simulink model "Simulink_Assignment2"  (R2020a)
settings: Solver=FixedStepAuto  StartTime=0.0  StopTime=10  FixedStep=1e-3  RelTol=1e-3  EnableMultiTasking=on
undefined symbols (not defined in the file): A0, A1, D0, D1, D10, D11, D12, D13, D2, D3, D4, D5, D6, D7, D8, D9, magnitude, PTA0, PTA1, PTA2, PTB2, PTB23, PTB3, PTB9, PTC16, PTC17, PTC2, PTC3, PTC4, PTD0, PTD1, PTD2, PTD3
libraries: frdmk64flib x19, etargetslib x8
settings Model: ExtModeTrigDuration=5  Creator=ryanb  LastModifiedBy=hunte
settings OptimizationCC: EnhancedBackFolding=on  PassReuseOutputArgsAs=Individual arguments  ZeroExternalMemoryAtStartup=off  ZeroInternalMemoryAtStartup=off  MaxStackSize=64  OptimizeBlockOrder=speed  DifferentSizesBufferReuse=on  OptimizationCustomize=off  EfficientTunableParamExpr=on
settings DebuggingCC: ParameterTunabilityLossMsg=error  UnconnectedInputMsg=none  UnconnectedOutputMsg=none  UnconnectedLineMsg=none
settings HardwareCC: ProdBitPerPointer=32  ProdBitPerSizeT=32  ProdBitPerPtrDiffT=32  ProdLargestAtomicInteger=Long  ProdLargestAtomicFloat=Double  ProdWordSize=32  ProdHWDeviceType=ARM Compatible->ARM Cortex
settings ModelReferenceCC: EnableRefExpFcnMdlSchedulingChecks=off
settings SFSimCC: MATLABDynamicMemAlloc=off
settings RTWCC: SystemTargetFile=ert.tlc  HardwareBoard=NXP FRDM-K64F  TemplateMakefile=ert_default_tmf  Toolchain=GNU Tools for ARM Embedded Processors
settings CodeAppCC: ForceParamTrailComments=on  IgnoreCustomStorageClasses=off  OperatorAnnotations=on  SimulinkDataObjDesc=on  SFDataObjDesc=on  InsertBlockDesc=on
settings ERTTargetCC: ExtModeTransport=4  ExtModeMexFile=sendToCommService

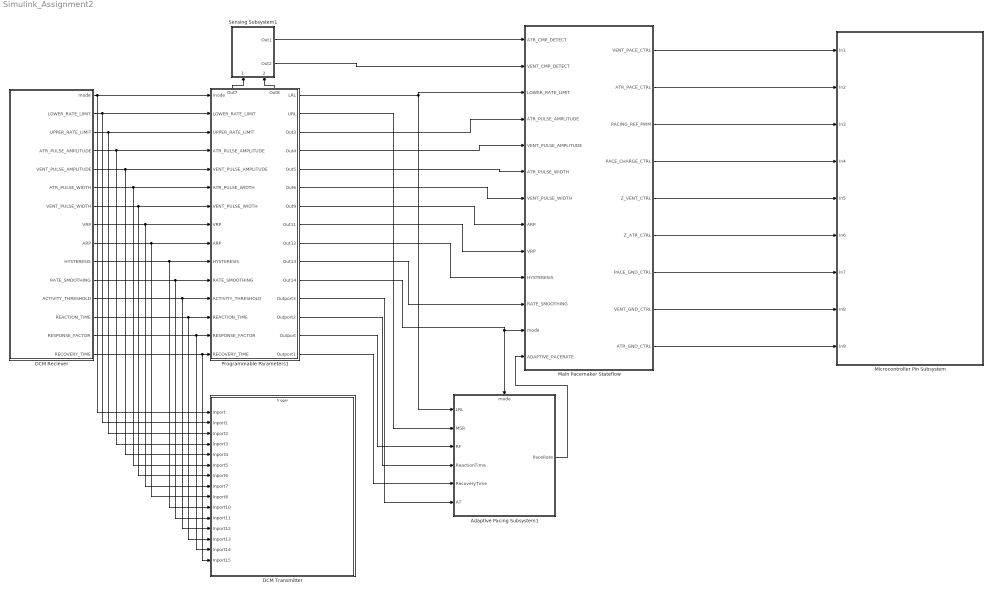
== system Simulink_Assignment2 ==
  Adaptive Pacing Subsystem1 : Subsystem
      settings: PortSchema="{\"entries\":[{\"content\":{\"sides\":[{\"content\":{\"connectorIds\":[\"In1\",\"In2\",\"In3\",\"In4\",\"In5\",\"In6\"]},\"type\":\"ConnectorPlacement.EquallySpacedRectSide\",\"uuid\":\"61dbb7e9-2003-4a43-93b8-10f5910df485\"},{\"content\":{\"connectorIds\":[\"Out1\"],\"side\":\"RIGHT\"},\"type\":\"ConnectorPlacement.EquallySpacedRectSide\",\"uuid\":\"cbb870a5-2f34-4900-b14d-ede4f510cea2\"},{\"content\":{\"connectorIds\":[\"In7\"],\"side\":\"TOP\"},\"type\":\"ConnectorPlacement.EquallySpacedRectSide\",\"uuid\":\"f277726d-3108-4a56-8fdd-1a2c1e5413e5\"}]},\"type\":\"ConnectorPlacement.EquallySpacedConnector\",\"uuid\":\"273ed509-6e25-4a7e-afb6-82e332976af3\"}],\"packageUris\":[\"http://schema.mathworks.com/mf0/Connector/R2020b\"],\"version\":\"1.0\"}"
  DCM Reciever : Subsystem
  DCM Transmitter : Subsystem
  Main Pacemaker Stateflow : Stateflow chart  TreatAsAtomicUnit=on
      settings: PortSchema="{\"entries\":[{\"content\":{\"sides\":[{\"content\":{\"connectorIds\":[\"In1\",\"In2\",\"In3\",\"In6\",\"In4\",\"In7\",\"In5\",\"In8\",\"In9\",\"In10\",\"In11\",\"In12\",\"In13\"]},\"type\":\"ConnectorPlacement.EquallySpacedRectSide\",\"uuid\":\"e04c6c9d-b568-4760-aae3-37103fc4b8a5\"},{\"content\":{\"connectorIds\":[\"Out1\",\"Out2\",\"Out3\",\"Out4\",\"Out5\",\"Out6\",\"Out7\",\"Out8\",\"Out9\"],\"side\":\"RIGHT\"},\"type\":\"ConnectorPlacement.EquallySpacedRectSide\",\"uuid\":\"410f5465-af00-4611-9887-c67099d36fd9\"},{\"content\":{\"connectorIds\":[],\"side\":\"TOP\"},\"type\":\"ConnectorPlacement.EquallySpacedRectSide\",\"uuid\":\"117107fa-ec70-4a57-9ea7-207f77d687e8\"}]},\"type\":\"ConnectorPlacement.EquallySpacedConnector\",\"uuid\":\"376840e9-6019-4e50-8c40-c1322fd1edca\"}],\"packageUris\":[\"http://schema.mathworks.com/mf0/Connector/19700101\"],\"version\":\"1.0\"}"
  Microcontroller Pin Subsystem : Subsystem
  Programmable Parameters1 : Subsystem
      settings: PortSchema="{\"entries\":[{\"content\":{\"sides\":[{\"content\":{\"connectorIds\":[\"In1\",\"In2\",\"In3\",\"In4\",\"In5\",\"In6\",\"In7\",\"In8\",\"In9\",\"In10\",\"In11\",\"In12\",\"In13\",\"In14\",\"In15\"]},\"type\":\"ConnectorPlacement.EquallySpacedRectSide\",\"uuid\":\"a66c8e23-13e5-4abc-9e09-ab5de47ab8f3\"},{\"content\":{\"connectorIds\":[\"Out1\",\"Out2\",\"Out3\",\"Out4\",\"Out5\",\"Out6\",\"Out7\",\"Out8\",\"Out9\",\"Out10\",\"Out11\",\"Out12\",\"Out13\",\"Out14\",\"Out15\"],\"side\":\"RIGHT\"},\"type\":\"ConnectorPlacement.EquallySpacedRectSide\",\"uuid\":\"6a9d25ad-44fc-45a2-8267-3a8c58854065\"},{\"content\":{\"connectorIds\":[\"Out16\",\"Out17\"],\"side\":\"TOP\"},\"type\":\"ConnectorPlacement.EquallySpacedRectSide\",\"uuid\":\"f44503e8-6d5f-481a-bd74-8db17b5d4837\"}]},\"type\":\"ConnectorPlacement.EquallySpacedConnector\",\"uuid\":\"c0ce9d52-7c52-4f4e-8e23-cf5f7806242f\"}],\"packageUris\":[\"http://schema.mathworks.com/mf0/Connector/19700101\"],\"version\":\"1.0\"}"
  Sensing Subsystem1 : Subsystem
      settings: PortSchema="{\"entries\":[{\"content\":{\"sides\":[{\"content\":{},\"type\":\"ConnectorPlacement.EquallySpacedRectSide\",\"uuid\":\"02e0911b-3253-486a-acb8-f1ba1f788aa5\"},{\"content\":{\"connectorIds\":[\"Out1\",\"Out2\"],\"side\":\"RIGHT\"},\"type\":\"ConnectorPlacement.EquallySpacedRectSide\",\"uuid\":\"66620bda-3110-4f43-a68e-d3775ac902e4\"},{\"content\":{\"side\":\"TOP\"},\"type\":\"ConnectorPlacement.EquallySpacedRectSide\",\"uuid\":\"5a7389cd-e024-434f-a78f-666a7db32550\"},{\"content\":{\"connectorIds\":[\"In1\",\"In2\"],\"side\":\"BOTTOM\"},\"type\":\"ConnectorPlacement.EquallySpacedRectSide\",\"uuid\":\"7cfc8cd2-653b-4c46-8563-1d8a50e07e7c\"}]},\"type\":\"ConnectorPlacement.EquallySpacedConnector\",\"uuid\":\"3e76420e-71f9-4267-bc59-506d487f0d17\"}],\"packageUris\":[\"http://schema.mathworks.com/mf0/Connector/R2020b\"],\"version\":\"1.0\"}"
  wires:
  Main Pacemaker Stateflow/1(VENT_PACE_CTRL) -> Microcontroller Pin Subsystem/1(In1)
  Main Pacemaker Stateflow/2(ATR_PACE_CTRL) -> Microcontroller Pin Subsystem/2(In2)
  Main Pacemaker Stateflow/3(PACING_REF_PWM) -> Microcontroller Pin Subsystem/3(In3)
  Main Pacemaker Stateflow/4(PACE_CHARGE_CTRL) -> Microcontroller Pin Subsystem/4(In4)
  Main Pacemaker Stateflow/5(Z_VENT_CTRL) -> Microcontroller Pin Subsystem/5(In5)
  Main Pacemaker Stateflow/6(Z_ATR_CTRL) -> Microcontroller Pin Subsystem/6(In6)
  Main Pacemaker Stateflow/7(PACE_GND_CTRL) -> Microcontroller Pin Subsystem/7(In7)
  Main Pacemaker Stateflow/8(VENT_GND_CTRL) -> Microcontroller Pin Subsystem/8(In8)
  Main Pacemaker Stateflow/9(ATR_GND_CTRL) -> Microcontroller Pin Subsystem/9(In9)
  DCM Reciever/15(RECOVERY_TIME) -> Programmable Parameters1/15(RECOVERY_TIME), DCM Transmitter/15(Inport15)
  DCM Reciever/2(LOWER_RATE_LIMIT) -> DCM Transmitter/2(Inport1), Programmable Parameters1/2(LOWER_RATE_LIMIT)
  DCM Reciever/1(mode) -> DCM Transmitter/1(Inport), Programmable Parameters1/1(mode)
  DCM Reciever/4(ATR_PULSE_AMPLITUDE) -> DCM Transmitter/4(Inport3), Programmable Parameters1/4(ATR_PULSE_AMPLITUDE)
  DCM Reciever/14(RESPONSE_FACTOR) -> Programmable Parameters1/14(RESPONSE_FACTOR), DCM Transmitter/14(Inport14)
  DCM Reciever/8(VRP) -> Programmable Parameters1/8(VRP), DCM Transmitter/8(Inport7)
  DCM Reciever/10(HYSTERESIS) -> DCM Transmitter/10(Inport10), Programmable Parameters1/10(HYSTERESIS)
  DCM Reciever/13(REACTION_TIME) -> Programmable Parameters1/13(REACTION_TIME), DCM Transmitter/13(Inport13)
  DCM Reciever/6(ATR_PULSE_WIDTH) -> Programmable Parameters1/6(ATR_PULSE_WIDTH), DCM Transmitter/6(Inport5)
  DCM Reciever/12(ACTIVITY_THRESHOLD) -> Programmable Parameters1/12(ACTIVITY_THRESHOLD), DCM Transmitter/12(Inport12)
  DCM Reciever/11(RATE_SMOOTHING) -> DCM Transmitter/11(Inport11), Programmable Parameters1/11(RATE_SMOOTHING)
  DCM Reciever/3(UPPER_RATE_LIMIT) -> DCM Transmitter/3(Inport2), Programmable Parameters1/3(UPPER_RATE_LIMIT)
  DCM Reciever/9(ARP) -> Programmable Parameters1/9(ARP), DCM Transmitter/9(Inport8)
  DCM Reciever/7(VENT_PULSE_WIDTH) -> Programmable Parameters1/7(VENT_PULSE_WIDTH), DCM Transmitter/7(Inport6)
  DCM Reciever/5(VENT_PULSE_AMPLITUDE) -> Programmable Parameters1/5(VENT_PULSE_AMPLITUDE), DCM Transmitter/5(Inport4)
  Programmable Parameters1/17(Out8) -> Sensing Subsystem1/2(ATR_SENSITIVITY)
  Programmable Parameters1/16(Out7) -> Sensing Subsystem1/1(VENT_SENSITIVITY)
  Sensing Subsystem1/1(Out1) -> Main Pacemaker Stateflow/1(ATR_CMP_DETECT)
  Sensing Subsystem1/2(Out2) -> Main Pacemaker Stateflow/2(VENT_CMP_DETECT)
  Programmable Parameters1/1(LRL) -> Main Pacemaker Stateflow/3(LOWER_RATE_LIMIT), Adaptive Pacing Subsystem1/1(LRL)
  Programmable Parameters1/7(Out9) -> Main Pacemaker Stateflow/8(ARP)
  Programmable Parameters1/3(Out3) -> Main Pacemaker Stateflow/6(ATR_PULSE_AMPLITUDE)
  Programmable Parameters1/4(Out4) -> Main Pacemaker Stateflow/4(VENT_PULSE_AMPLITUDE)
  Programmable Parameters1/5(Out5) -> Main Pacemaker Stateflow/7(ATR_PULSE_WIDTH)
  Programmable Parameters1/6(Out6) -> Main Pacemaker Stateflow/5(VENT_PULSE_WIDTH)
  Programmable Parameters1/8(Out11) -> Main Pacemaker Stateflow/9(VRP)
  Programmable Parameters1/9(Out12) -> Main Pacemaker Stateflow/10(HYSTERESIS)
  Programmable Parameters1/10(Out13) -> Main Pacemaker Stateflow/11(RATE_SMOOTHING)
  Programmable Parameters1/11(Out14) -> Adaptive Pacing Subsystem1/7(mode), Main Pacemaker Stateflow/12(mode)
  Programmable Parameters1/14(Outport) -> Adaptive Pacing Subsystem1/3(RF)
  Programmable Parameters1/13(Outport2) -> Adaptive Pacing Subsystem1/4(ReactionTime)
  Programmable Parameters1/15(Outport1) -> Adaptive Pacing Subsystem1/5(RecoveryTime)
  Programmable Parameters1/12(Outport3) -> Adaptive Pacing Subsystem1/6(AT)
  Adaptive Pacing Subsystem1/1(PaceRate) -> Main Pacemaker Stateflow/13(ADAPTIVE_PACERATE)
  Programmable Parameters1/2(URL) -> Adaptive Pacing Subsystem1/2(MSR)

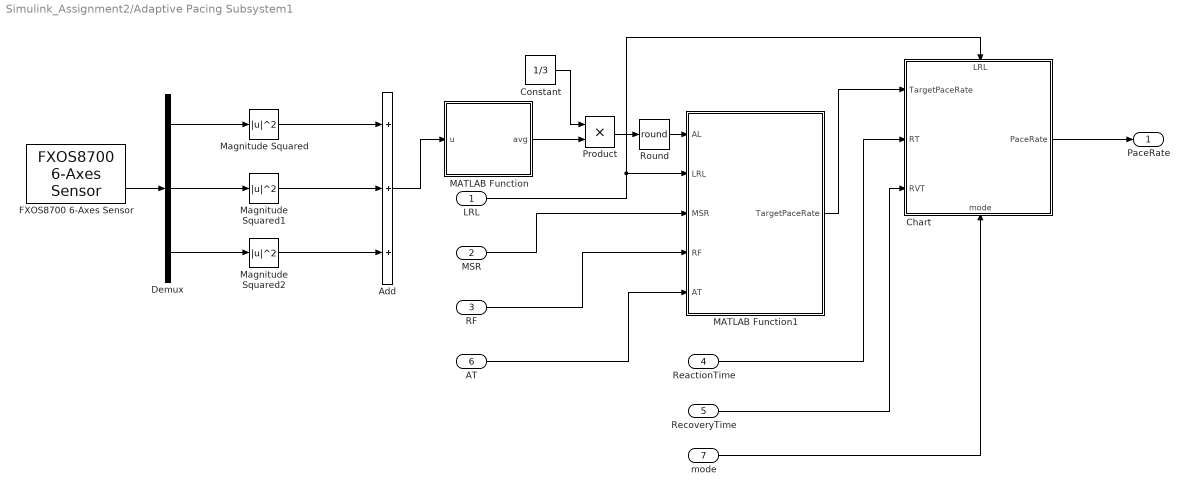
== system Simulink_Assignment2/Adaptive Pacing Subsystem1 ==
  LRL : Inport
  MSR : Inport  Port=2
  RF : Inport  Port=3
  ReactionTime : Inport  Port=4
  RecoveryTime : Inport  Port=5
  AT : Inport  Port=6
  mode : Inport  Port=7
  Add : Sum  Inputs=+++
  Chart : Stateflow chart  TreatAsAtomicUnit=on
      settings: PortSchema="{\"entries\":[{\"content\":{\"sides\":[{\"content\":{\"connectorIds\":[\"In4\",\"In5\",\"In3\"]},\"type\":\"ConnectorPlacement.EquallySpacedRectSide\",\"uuid\":\"73e2e136-6579-428c-8934-f1198b959902\"},{\"content\":{\"connectorIds\":[\"Out1\"],\"side\":\"RIGHT\"},\"type\":\"ConnectorPlacement.EquallySpacedRectSide\",\"uuid\":\"2b83c2c9-79e9-4b77-8584-7bf14575e11f\"},{\"content\":{\"connectorIds\":[\"In2\"],\"side\":\"TOP\"},\"type\":\"ConnectorPlacement.EquallySpacedRectSide\",\"uuid\":\"a1e24dee-acf3-4d04-b3f5-e7985e86027f\"},{\"content\":{\"connectorIds\":[\"In1\"],\"side\":\"BOTTOM\"},\"type\":\"ConnectorPlacement.EquallySpacedRectSide\",\"uuid\":\"104b9065-8074-4090-9dc5-4a66f5aa0eec\"}]},\"type\":\"ConnectorPlacement.EquallySpacedConnector\",\"uuid\":\"c053058d-9bc6-48c2-85b3-1dbac630ff6a\"}],\"packageUris\":[\"http://schema.mathworks.com/mf0/Connector/R2020b\"],\"version\":\"1.0\"}"
  Constant : Constant  Value=1/3
  Demux : Demux  Outputs=3
  FXOS8700 6-Axes Sensor : frdmk64flib/FXOS8700 6-Axes Sensor  Activesensor=Accelerometer and Magnetometer  ODR=800Hz  HybridODR=200Hz  Accelfullrange=-4g to +4g  SampleTime=-1
  MATLAB Function : MATLAB Function  TreatAsAtomicUnit=on
  MATLAB Function1 : MATLAB Function  TreatAsAtomicUnit=on
  Magnitude Squared : Math  Operator=magnitude^2  SaturateOnIntegerOverflow=on
  Magnitude Squared1 : Math  Operator=magnitude^2  SaturateOnIntegerOverflow=on
  Magnitude Squared2 : Math  Operator=magnitude^2  SaturateOnIntegerOverflow=on
  Product : Product
  Round : Rounding  Operator=round
  PaceRate : Outport
  wires:
  Add/1 -> MATLAB Function/1(u)
  LRL/1 -> Chart/2(LRL), MATLAB Function1/2(LRL)
  Demux/1 -> Magnitude Squared/1
  Magnitude Squared1/1 -> Add/2
  ReactionTime/1 -> Chart/5(RT)
  MSR/1 -> MATLAB Function1/3(MSR)
  Demux/3 -> Magnitude Squared2/1
  Magnitude Squared/1 -> Add/1
  Magnitude Squared2/1 -> Add/3
  Demux/2 -> Magnitude Squared1/1
  MATLAB Function1/1(TargetPaceRate) -> Chart/4(TargetPaceRate)
  Chart/1(PaceRate) -> PaceRate/1
  RecoveryTime/1 -> Chart/3(RVT)
  mode/1 -> Chart/1(mode)
  MATLAB Function/1(avg) -> Product/2
  Constant/1 -> Product/1
  Product/1 -> Round/1
  Round/1 -> MATLAB Function1/1(AL)
  RF/1 -> MATLAB Function1/4(RF)
  AT/1 -> MATLAB Function1/5(AT)
  FXOS8700 6-Axes Sensor/2 -> Demux/1

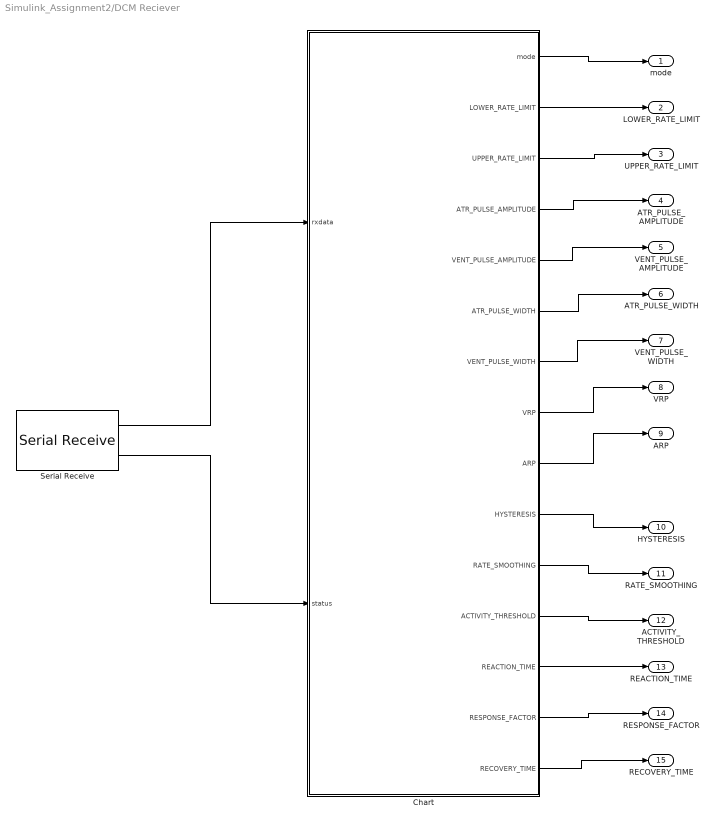
== system Simulink_Assignment2/DCM Reciever ==
  Chart : Stateflow chart  TreatAsAtomicUnit=on
      settings: PortSchema="{\"entries\":[{\"content\":{\"sides\":[{\"content\":{\"connectorIds\":[\"In2\",\"In1\"]},\"type\":\"ConnectorPlacement.EquallySpacedRectSide\",\"uuid\":\"86a0e5b4-c807-4287-9f41-a7f218213397\"},{\"content\":{\"connectorIds\":[\"Out1\",\"Out2\",\"Out3\",\"Out4\",\"Out5\",\"Out6\",\"Out7\",\"Out8\",\"Out9\",\"Out10\",\"Out11\",\"Out12\",\"Out13\",\"Out14\",\"Out15\"],\"side\":\"RIGHT\"},\"type\":\"ConnectorPlacement.EquallySpacedRectSide\",\"uuid\":\"103aaf26-9f93-4347-8cdc-d8dec7ff725b\"},{\"content\":{\"connectorIds\":[],\"side\":\"TOP\"},\"type\":\"ConnectorPlacement.EquallySpacedRectSide\",\"uuid\":\"6f19ed7d-8feb-4f02-b534-280b851845bc\"}]},\"type\":\"ConnectorPlacement.EquallySpacedConnector\",\"uuid\":\"a620034f-9c63-474d-a92f-595da83135da\"}],\"packageUris\":[\"http://schema.mathworks.com/mf0/Connector/19700101\"],\"version\":\"1.0\"}"
  Serial Receive : frdmk64flib/Serial Receive  SCIModule=0  Baudrate=uint32(9600)  Parity=None  StopBits=1  HardwareFlowControl=None  ByteOrder=LittleEndian  DataType=uint8  DataLength=31  BlockingMode=off  OutputStatus=on  SampleTime=-1
  mode : Outport
  LOWER_RATE_LIMIT : Outport  Port=2
  UPPER_RATE_LIMIT : Outport  Port=3
  ATR_PULSE_AMPLITUDE : Outport  Port=4
  VENT_PULSE_AMPLITUDE : Outport  Port=5
  ATR_PULSE_WIDTH : Outport  Port=6
  VENT_PULSE_WIDTH : Outport  Port=7
  VRP : Outport  Port=8
  ARP : Outport  Port=9
  HYSTERESIS : Outport  Port=10
  RATE_SMOOTHING : Outport  Port=11
  ACTIVITY_THRESHOLD : Outport  Port=12
  REACTION_TIME : Outport  Port=13
  RESPONSE_FACTOR : Outport  Port=14
  RECOVERY_TIME : Outport  Port=15
  wires:
  Serial Receive/1 -> Chart/2(rxdata)
  Serial Receive/2 -> Chart/1(status)
  Chart/1(mode) -> mode/1
  Chart/2(LOWER_RATE_LIMIT) -> LOWER_RATE_LIMIT/1
  Chart/3(UPPER_RATE_LIMIT) -> UPPER_RATE_LIMIT/1
  Chart/4(ATR_PULSE_AMPLITUDE) -> ATR_PULSE_AMPLITUDE/1
  Chart/5(VENT_PULSE_AMPLITUDE) -> VENT_PULSE_AMPLITUDE/1
  Chart/6(ATR_PULSE_WIDTH) -> ATR_PULSE_WIDTH/1
  Chart/7(VENT_PULSE_WIDTH) -> VENT_PULSE_WIDTH/1
  Chart/8(VRP) -> VRP/1
  Chart/9(ARP) -> ARP/1
  Chart/10(HYSTERESIS) -> HYSTERESIS/1
  Chart/11(RATE_SMOOTHING) -> RATE_SMOOTHING/1
  Chart/12(ACTIVITY_THRESHOLD) -> ACTIVITY_THRESHOLD/1
  Chart/13(REACTION_TIME) -> REACTION_TIME/1
  Chart/14(RESPONSE_FACTOR) -> RESPONSE_FACTOR/1
  Chart/15(RECOVERY_TIME) -> RECOVERY_TIME/1

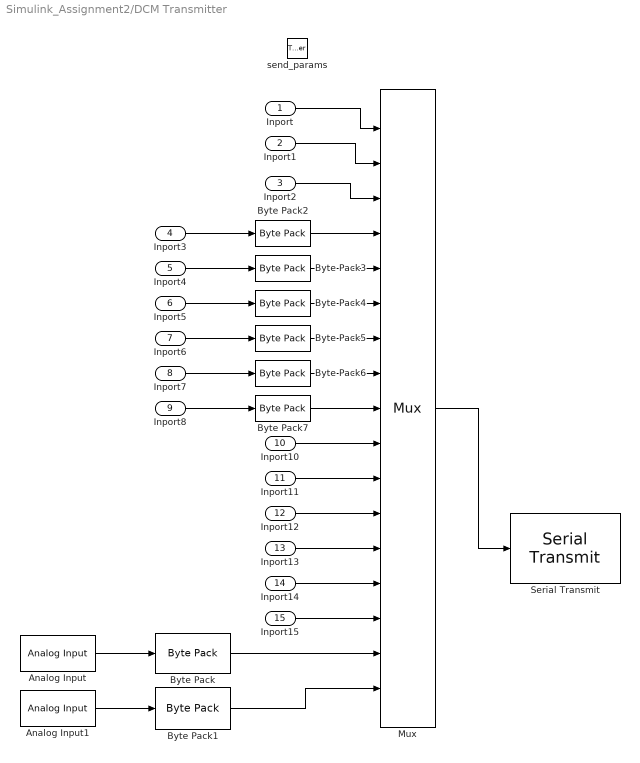
== system Simulink_Assignment2/DCM Transmitter ==
  Inport : Inport
  Inport1 : Inport  Port=2
  Inport2 : Inport  Port=3
  Inport3 : Inport  Port=4
  Inport4 : Inport  Port=5
  Inport5 : Inport  Port=6
  Inport6 : Inport  Port=7
  Inport7 : Inport  Port=8
  Inport8 : Inport  Port=9
  Inport10 : Inport  Port=10
  Inport11 : Inport  Port=11
  Inport12 : Inport  Port=12
  Inport13 : Inport  Port=13
  Inport14 : Inport  Port=14
  Inport15 : Inport  Port=15
  send_params : TriggerPort  TriggerType=function-call  IsSimulinkFunction=on  FunctionName=send_params  VariantControl=Variant  PortDimensions=1
  Analog Input : frdmk64flib/Analog Input  Whichpin=PTB2 (A0)  SampleTime=-1
  Analog Input1 : frdmk64flib/Analog Input  Whichpin=PTB3 (A1)  SampleTime=-1
  Byte Pack : etargetslib/Byte Pack  datatypes={'double'}  byteAlign=1
  Byte Pack1 : etargetslib/Byte Pack  datatypes={'double'}  byteAlign=1
  Byte Pack{2..5} (4 alike) : etargetslib/Byte Pack  datatypes={'single'}  byteAlign=1
  Byte Pack6 : etargetslib/Byte Pack  datatypes={'uint16'}  byteAlign=1
  Byte Pack7 : etargetslib/Byte Pack  datatypes={'uint16'}  byteAlign=1
  Mux : Mux  Inputs=17
  Serial Transmit : frdmk64flib/Serial Transmit  SCIModule=0  Baudrate=uint32(9600)  Parity=None  StopBits=1  HardwareFlowControl=None  ByteOrder=LittleEndian  BlockingMode=on  OutputStatus=off
  wires:
  Analog Input/1 -> Byte Pack/1
  Analog Input1/1 -> Byte Pack1/1
  Byte Pack1/1 -> Mux/17
  Byte Pack/1 -> Mux/16
  Mux/1 -> Serial Transmit/1
  Inport/1 -> Mux/1
  Inport1/1 -> Mux/2
  Inport2/1 -> Mux/3
  Inport14/1 -> Mux/14
  Inport15/1 -> Mux/15
  Inport13/1 -> Mux/13
  Inport12/1 -> Mux/12
  Inport11/1 -> Mux/11
  Inport10/1 -> Mux/10
  Inport3/1 -> Byte Pack2/1
  Byte Pack2/1 -> Mux/4
  Inport4/1 -> Byte Pack3/1
  Byte Pack3/1 -> Mux/5
  Inport5/1 -> Byte Pack4/1
  Byte Pack4/1 -> Mux/6
  Inport6/1 -> Byte Pack5/1
  Byte Pack5/1 -> Mux/7
  Inport7/1 -> Byte Pack6/1
  Byte Pack6/1 -> Mux/8
  Inport8/1 -> Byte Pack7/1
  Byte Pack7/1 -> Mux/9

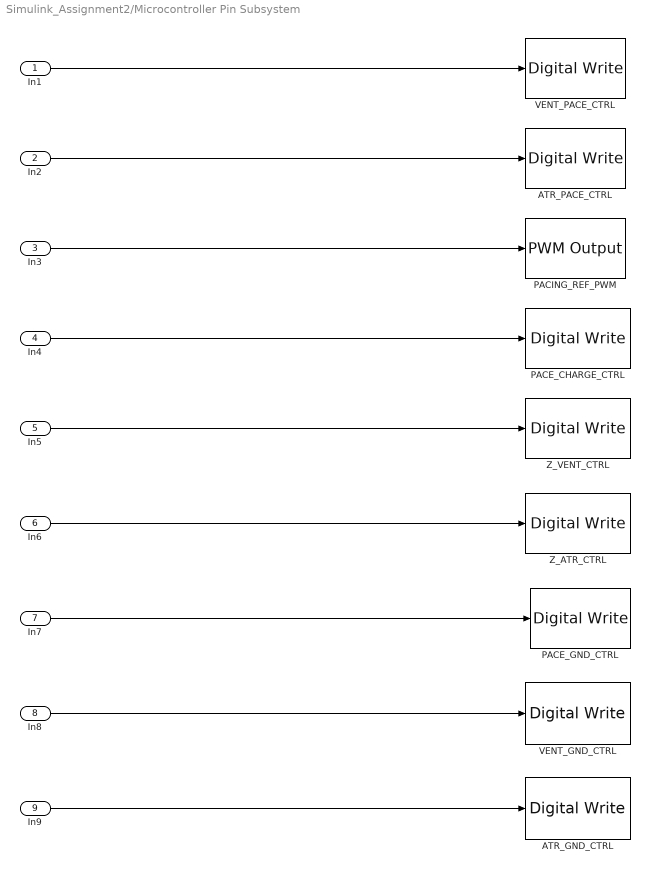
== system Simulink_Assignment2/Microcontroller Pin Subsystem ==
  In1 : Inport
  In2 : Inport  Port=2
  In3 : Inport  Port=3
  In4 : Inport  Port=4
  In5 : Inport  Port=5
  In6 : Inport  Port=6
  In7 : Inport  Port=7
  In8 : Inport  Port=8
  In9 : Inport  Port=9
  ATR_GND_CTRL : frdmk64flib/Digital Write  Whichpin=PTD2 (D11)
  ATR_PACE_CTRL : frdmk64flib/Digital Write  Whichpin=PTA0 (D8)
  PACE_CHARGE_CTRL : frdmk64flib/Digital Write  Whichpin=PTB9 (D2)
  PACE_GND_CTRL : frdmk64flib/Digital Write  Whichpin=PTD0 (D10)
  PACING_REF_PWM : frdmk64flib/PWM Output  Whichpin=PTA2 (D5)  InitialFrequency=2000  InitialDutyCycle=0
  VENT_GND_CTRL : frdmk64flib/Digital Write  Whichpin=PTD3 (D12)
  VENT_PACE_CTRL : frdmk64flib/Digital Write  Whichpin=PTC4 (D9)
  Z_ATR_CTRL : frdmk64flib/Digital Write  Whichpin=PTB23 (D4)
  Z_VENT_CTRL : frdmk64flib/Digital Write  Whichpin=PTC3 (D7)
  wires:
  In5/1 -> Z_VENT_CTRL/1
  In2/1 -> ATR_PACE_CTRL/1
  In6/1 -> Z_ATR_CTRL/1
  In8/1 -> VENT_GND_CTRL/1
  In4/1 -> PACE_CHARGE_CTRL/1
  In7/1 -> PACE_GND_CTRL/1
  In3/1 -> PACING_REF_PWM/1
  In1/1 -> VENT_PACE_CTRL/1
  In9/1 -> ATR_GND_CTRL/1

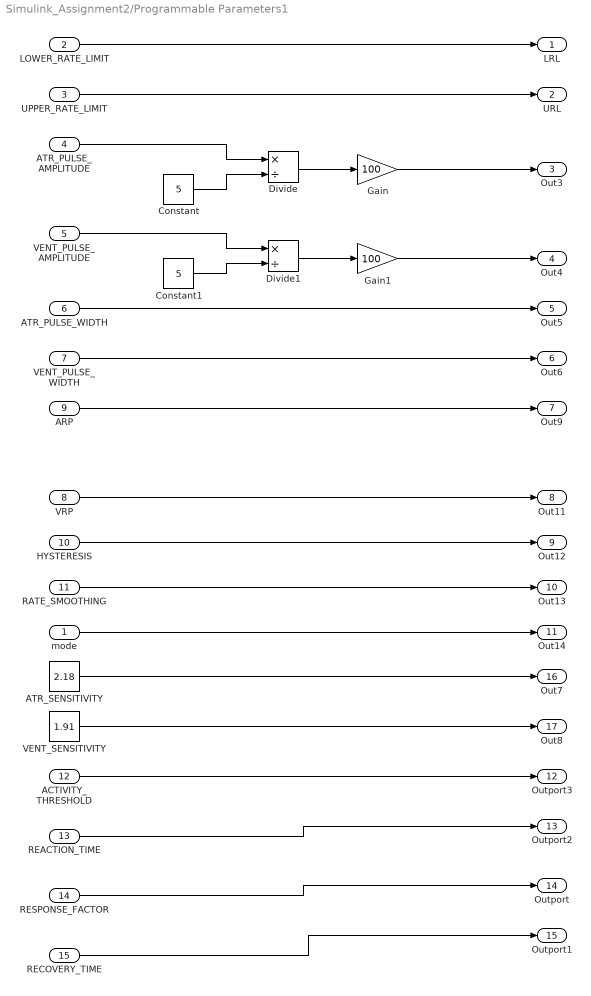
== system Simulink_Assignment2/Programmable Parameters1 ==
  mode : Inport
  LOWER_RATE_LIMIT : Inport  Port=2
  UPPER_RATE_LIMIT : Inport  Port=3
  ATR_PULSE_AMPLITUDE : Inport  Port=4
  VENT_PULSE_AMPLITUDE : Inport  Port=5
  ATR_PULSE_WIDTH : Inport  Port=6
  VENT_PULSE_WIDTH : Inport  Port=7
  VRP : Inport  Port=8
  ARP : Inport  Port=9
  HYSTERESIS : Inport  Port=10
  RATE_SMOOTHING : Inport  Port=11
  ACTIVITY_THRESHOLD : Inport  Port=12
  REACTION_TIME : Inport  Port=13
  RESPONSE_FACTOR : Inport  Port=14
  RECOVERY_TIME : Inport  Port=15
  ATR_SENSITIVITY : Constant  Value=2.18
  Constant : Constant  Value=5
  Constant1 : Constant  Value=5
  Divide : Product  Inputs=*/
  Divide1 : Product  Inputs=*/
  Gain : Gain  Gain=100
  Gain1 : Gain  Gain=100
  VENT_SENSITIVITY : Constant  Value=1.91
  LRL : Outport
  URL : Outport  Port=2
  Out3 : Outport  Port=3
  Out4 : Outport  Port=4
  Out5 : Outport  Port=5
  Out6 : Outport  Port=6
  Out9 : Outport  Port=7
  Out11 : Outport  Port=8
  Out12 : Outport  Port=9
  Out13 : Outport  Port=10
  Out14 : Outport  Port=11
  Outport3 : Outport  Port=12
  Outport2 : Outport  Port=13
  Outport : Outport  Port=14
  Outport1 : Outport  Port=15
  Out7 : Outport  Port=16
  Out8 : Outport  Port=17
  wires:
  VENT_SENSITIVITY/1 -> Out8/1
  HYSTERESIS/1 -> Out12/1
  ATR_SENSITIVITY/1 -> Out7/1
  ARP/1 -> Out9/1
  VRP/1 -> Out11/1
  RATE_SMOOTHING/1 -> Out13/1
  UPPER_RATE_LIMIT/1 -> URL/1
  LOWER_RATE_LIMIT/1 -> LRL/1
  ATR_PULSE_AMPLITUDE/1 -> Divide/1
  Constant/1 -> Divide/2
  VENT_PULSE_AMPLITUDE/1 -> Divide1/1
  Constant1/1 -> Divide1/2
  Gain/1 -> Out3/1
  Divide/1 -> Gain/1
  Divide1/1 -> Gain1/1
  Gain1/1 -> Out4/1
  ATR_PULSE_WIDTH/1 -> Out5/1
  VENT_PULSE_WIDTH/1 -> Out6/1
  mode/1 -> Out14/1
  ACTIVITY_THRESHOLD/1 -> Outport3/1
  REACTION_TIME/1 -> Outport2/1
  RESPONSE_FACTOR/1 -> Outport/1
  RECOVERY_TIME/1 -> Outport1/1

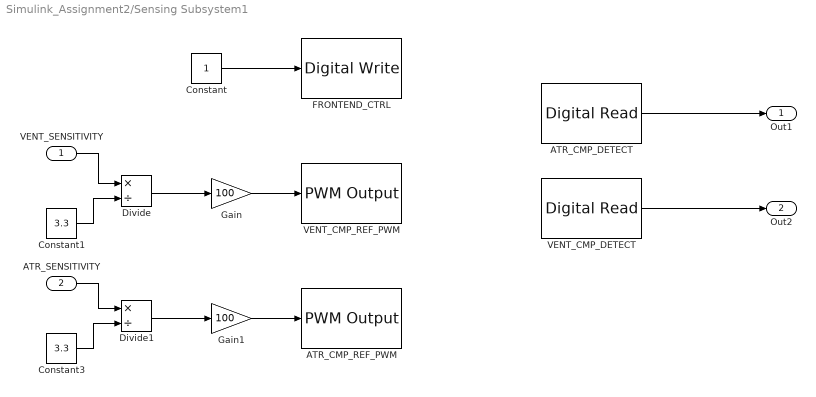
== system Simulink_Assignment2/Sensing Subsystem1 ==
  VENT_SENSITIVITY : Inport
  ATR_SENSITIVITY : Inport  Port=2
  ATR_CMP_DETECT : frdmk64flib/Digital Read  Whichpin=PTC16 (D0)  SampleTime=-1
  ATR_CMP_REF_PWM : frdmk64flib/PWM Output  Whichpin=PTC2 (D6)  InitialFrequency=2000  InitialDutyCycle=0
  Constant : Constant
  Constant1 : Constant  Value=3.3
  Constant3 : Constant  Value=3.3
  Divide : Product  Inputs=*/
  Divide1 : Product  Inputs=*/
  FRONTEND_CTRL : frdmk64flib/Digital Write  Whichpin=PTD1 (D13)
  Gain : Gain  Gain=100
  Gain1 : Gain  Gain=100
  VENT_CMP_DETECT : frdmk64flib/Digital Read  Whichpin=PTC17 (D1)  SampleTime=-1
  VENT_CMP_REF_PWM : frdmk64flib/PWM Output  Whichpin=PTA1 (D3)  InitialFrequency=2000  InitialDutyCycle=0
  Out1 : Outport
  Out2 : Outport  Port=2
  wires:
  VENT_CMP_DETECT/1 -> Out2/1
  ATR_CMP_DETECT/1 -> Out1/1
  VENT_SENSITIVITY/1 -> Divide/1
  Constant1/1 -> Divide/2
  Constant3/1 -> Divide1/2
  ATR_SENSITIVITY/1 -> Divide1/1
  Gain1/1 -> ATR_CMP_REF_PWM/1
  Gain/1 -> VENT_CMP_REF_PWM/1
  Divide/1 -> Gain/1
  Divide1/1 -> Gain1/1
  Constant/1 -> FRONTEND_CTRL/1

== stateflow chart Simulink_Assignment2/Main Pacemaker Stateflow ==
  state Startup
  state VOO
    state PACING
      entry:
      PACE_CHARGE_CTRL = 0;
      PACE_GND_CTRL = 1;
      ATR_PACE_CTRL = 0;
      ATR_GND_CTRL = 0;
      Z_ATR_CTRL = 0;
      Z_VENT_CTRL = 0;
      VENT_GND_CTRL = 0;
      VENT_PACE_CTRL = 1;
    state CHARGING
      entry:
      %%Charging C22
      ATR_PACE_CTRL = 0;
      VENT_PACE_CTRL = 0;
      PACE_CHARGE_CTRL = 1;
      %%Discharging Blocking Cap
      PACE_GND_CTRL = 1;
      Z_ATR_CTRL = 0;
      Z_VENT_CTRL = 0;
      ATR_GND_CTRL = 0;
      VENT_GND_CTRL = 1;
      PACING_REF_PWM = VENT_PULSE_AMPLITUDE;
    VOO.CHARGING -> VOO.PACING [order 2] : %%Pace Ready
        | [after(1/(double(LOWER_RATE_LIMIT)/60000) - double(VENT_PULSE_WIDTH), msec)]
    VOO.PACING -> VOO.CHARGING : %%Recharge Ready
        | [after(VENT_PULSE_WIDTH, msec)]
  state AOO
    state PACING
      entry:
      PACE_CHARGE_CTRL = 0;
      PACE_GND_CTRL = 1;
      ATR_PACE_CTRL = 1;
      ATR_GND_CTRL = 0;
      Z_ATR_CTRL = 0;
      Z_VENT_CTRL = 0;
      VENT_GND_CTRL = 0;
      VENT_PACE_CTRL = 0;
    state CHARGING
      entry:
      %%Charging C22
      ATR_PACE_CTRL = 0;
      VENT_PACE_CTRL = 0;
      PACE_CHARGE_CTRL = 1;
      %%Discharging Blocking Cap
      PACE_GND_CTRL = 1;
      Z_ATR_CTRL = 0;
      Z_VENT_CTRL = 0;
      ATR_GND_CTRL = 1;
      VENT_GND_CTRL = 0;
      PACING_REF_PWM = ATR_PULSE_AMPLITUDE;
    AOO.CHARGING -> AOO.PACING [order 1] : %%Pace Ready
        | [after(1/(double(LOWER_RATE_LIMIT)/60000) - double(ATR_PULSE_WIDTH), msec)]
    AOO.PACING -> AOO.CHARGING : %%Recharge Ready
        | [after(ATR_PULSE_WIDTH, msec)]
  state VVI
    state CHARGING
      entry:
      %%Charging C22
      ATR_PACE_CTRL = 0;
      VENT_PACE_CTRL = 0;
      PACE_CHARGE_CTRL = 1;
      %%Discharging Blocking Cap
      PACE_GND_CTRL = 1;
      Z_ATR_CTRL = 0;
      Z_VENT_CTRL = 0;
      ATR_GND_CTRL = 0;
      VENT_GND_CTRL = 1;
      PACING_REF_PWM = VENT_PULSE_AMPLITUDE;
    state PACING
      entry:
      PACE_CHARGE_CTRL = 0;
      PACE_GND_CTRL = 1;
      ATR_PACE_CTRL = 0;
      ATR_GND_CTRL = 0;
      Z_ATR_CTRL = 0;
      Z_VENT_CTRL = 0;
      VENT_GND_CTRL = 0;
      VENT_PACE_CTRL = 1;
    (junction 128) -> VVI.PACING [order 1] : %%Pace Ready
        | [after(1/(double(LOWER_RATE_LIMIT)/60000) - double(VENT_PULSE_WIDTH) - VRP, msec) && VENT_CMP_DETECT == false]
    VVI.CHARGING -> (junction 128) [order 1] : [after(VRP, msec)]
    (junction 128) -> VVI.CHARGING [order 2] : [VENT_CMP_DETECT == true]
    VVI.PACING -> VVI.CHARGING : [after(VENT_PULSE_WIDTH, msec)]
  state AAI
    state PACING
      entry:
      PACE_CHARGE_CTRL = 0;
      PACE_GND_CTRL = 1;
      ATR_PACE_CTRL = 1;
      ATR_GND_CTRL = 0;
      Z_ATR_CTRL = 0;
      Z_VENT_CTRL = 0;
      VENT_GND_CTRL = 0;
      VENT_PACE_CTRL = 0;
    state CHARGING
      entry:
      %%Charging C22
      ATR_PACE_CTRL = 0;
      VENT_PACE_CTRL = 0;
      PACE_CHARGE_CTRL = 1;
      %%Discharging Blocking Cap
      PACE_GND_CTRL = 1;
      Z_ATR_CTRL = 0;
      Z_VENT_CTRL = 0;
      ATR_GND_CTRL = 1;
      VENT_GND_CTRL = 0;
      PACING_REF_PWM = ATR_PULSE_AMPLITUDE;
    (junction 142) -> AAI.PACING [order 1] : %%Pace Ready
        | [after(1/(double(LOWER_RATE_LIMIT)/60000) - double(ATR_PULSE_WIDTH) - ARP, msec) && ATR_CMP_DETECT == false]
    AAI.CHARGING -> (junction 142) [order 1] : [after(ARP, msec)]
    (junction 142) -> AAI.CHARGING [order 2] : [ATR_CMP_DETECT == true]
    AAI.PACING -> AAI.CHARGING : %%Recharge Ready
        | [after(ATR_PULSE_WIDTH, msec)]
  state AOOR
    state PACING
      entry:
      PACE_CHARGE_CTRL = 0;
      PACE_GND_CTRL = 1;
      ATR_PACE_CTRL = 1;
      ATR_GND_CTRL = 0;
      Z_ATR_CTRL = 0;
      Z_VENT_CTRL = 0;
      VENT_GND_CTRL = 0;
      VENT_PACE_CTRL = 0;
    state CHARGING
      entry:
      %%Charging C22
      ATR_PACE_CTRL = 0;
      VENT_PACE_CTRL = 0;
      PACE_CHARGE_CTRL = 1;
      %%Discharging Blocking Cap
      PACE_GND_CTRL = 1;
      Z_ATR_CTRL = 0;
      Z_VENT_CTRL = 0;
      ATR_GND_CTRL = 1;
      VENT_GND_CTRL = 0;
      PACING_REF_PWM = ATR_PULSE_AMPLITUDE;
    AOOR.CHARGING -> AOOR.PACING [order 1] : %%Pace Ready
        | [after(1/(double(ADAPTIVE_PACERATE)/60000) - double(ATR_PULSE_WIDTH), msec)]
    AOOR.PACING -> AOOR.CHARGING : %%Recharge Ready
        | [after(ATR_PULSE_WIDTH, msec)]
  state VOOR
    state PACING
      entry:
      PACE_CHARGE_CTRL = 0;
      PACE_GND_CTRL = 1;
      ATR_PACE_CTRL = 0;
      ATR_GND_CTRL = 0;
      Z_ATR_CTRL = 0;
      Z_VENT_CTRL = 0;
      VENT_GND_CTRL = 0;
      VENT_PACE_CTRL = 1;
    state CHARGING
      entry:
      %%Charging C22
      ATR_PACE_CTRL = 0;
      VENT_PACE_CTRL = 0;
      PACE_CHARGE_CTRL = 1;
      %%Discharging Blocking Cap
      PACE_GND_CTRL = 1;
      Z_ATR_CTRL = 0;
      Z_VENT_CTRL = 0;
      ATR_GND_CTRL = 0;
      VENT_GND_CTRL = 1;
      PACING_REF_PWM = VENT_PULSE_AMPLITUDE;
    VOOR.CHARGING -> VOOR.PACING [order 2] : %%Pace Ready
        | [after(1/(double(ADAPTIVE_PACERATE)/60000) - double(VENT_PULSE_WIDTH), msec)]
    VOOR.PACING -> VOOR.CHARGING : %%Recharge Ready
        | [after(VENT_PULSE_WIDTH, msec)]
  state AAIR
    state PACING
      entry:
      PACE_CHARGE_CTRL = 0;
      PACE_GND_CTRL = 1;
      ATR_PACE_CTRL = 1;
      ATR_GND_CTRL = 0;
      Z_ATR_CTRL = 0;
      Z_VENT_CTRL = 0;
      VENT_GND_CTRL = 0;
      VENT_PACE_CTRL = 0;
    state CHARGING
      entry:
      %%Charging C22
      ATR_PACE_CTRL = 0;
      VENT_PACE_CTRL = 0;
      PACE_CHARGE_CTRL = 1;
      %%Discharging Blocking Cap
      PACE_GND_CTRL = 1;
      Z_ATR_CTRL = 0;
      Z_VENT_CTRL = 0;
      ATR_GND_CTRL = 1;
      VENT_GND_CTRL = 0;
      PACING_REF_PWM = ATR_PULSE_AMPLITUDE;
    (junction 175) -> AAIR.PACING [order 1] : %%Pace Ready
        | [after(1/(double(ADAPTIVE_PACERATE)/60000) - double(ATR_PULSE_WIDTH) - ARP, msec) && ATR_CMP_DETECT == false]
    AAIR.CHARGING -> (junction 175) [order 1] : [after(ARP, msec)]
    (junction 175) -> AAIR.CHARGING [order 2] : [ATR_CMP_DETECT == true]
    AAIR.PACING -> AAIR.CHARGING : %%Recharge Ready
        | [after(ATR_PULSE_WIDTH, msec)]
  state VVIR
    state PACING
      entry:
      PACE_CHARGE_CTRL = 0;
      PACE_GND_CTRL = 1;
      ATR_PACE_CTRL = 0;
      ATR_GND_CTRL = 0;
      Z_ATR_CTRL = 0;
      Z_VENT_CTRL = 0;
      VENT_GND_CTRL = 0;
      VENT_PACE_CTRL = 1;
    state CHARGING
      entry:
      %%Charging C22
      ATR_PACE_CTRL = 0;
      VENT_PACE_CTRL = 0;
      PACE_CHARGE_CTRL = 1;
      %%Discharging Blocking Cap
      PACE_GND_CTRL = 1;
      Z_ATR_CTRL = 0;
      Z_VENT_CTRL = 0;
      ATR_GND_CTRL = 0;
      VENT_GND_CTRL = 1;
      PACING_REF_PWM = ATR_PULSE_AMPLITUDE;
    (junction 186) -> VVIR.PACING [order 1] : %%Pace Ready
        | [after(1/(double(ADAPTIVE_PACERATE)/60000) - double(VENT_PULSE_WIDTH) - VRP, msec) && VENT_CMP_DETECT == false]
    VVIR.CHARGING -> (junction 186) [order 1] : [after(VRP, msec)]
    (junction 186) -> VVIR.CHARGING [order 2] : [VENT_CMP_DETECT == true]
    VVIR.PACING -> VVIR.CHARGING : %%Recharge Ready
        | [after(VENT_PULSE_WIDTH, msec)]
  Startup -> AOOR.CHARGING [order 5] : [mode == 5]
  Startup -> VOOR.CHARGING [order 6] : [mode == 6]
  Startup -> AAIR.CHARGING [order 7] : [mode == 7]
  Startup -> VVIR.CHARGING [order 8] : [mode == 8]
  AAIR.CHARGING -> Startup [order 2] : [mode ~= 7]
  VVIR.CHARGING -> Startup [order 2] : [mode ~= 8]
  AAI.CHARGING -> Startup [order 2] : [mode ~= 4]
  AOO.CHARGING -> Startup [order 2] : [mode ~= 2]
  VVI.CHARGING -> Startup [order 2] : [mode ~= 3]
  Startup -> VOO.CHARGING [order 4] : [mode == 1]
  AOOR.CHARGING -> Startup [order 2] : [mode ~= 5]
  VOO.CHARGING -> Startup [order 1] : [mode ~= 1]
  VOOR.CHARGING -> Startup [order 1] : [mode ~= 6]
  (default) -> Startup
  Startup -> AOO.CHARGING [order 1] : [mode == 2]
  Startup -> VVI.CHARGING [order 2] : [mode == 3]
  Startup -> AAI.CHARGING [order 3] : [mode == 4]
  Startup -> Startup [order 9] : [mode == 9]
  data: ATR_CMP_DETECT input; VENT_CMP_DETECT input; VENT_PACE_CTRL output; ATR_PACE_CTRL output; PACING_REF_PWM output; PACE_CHARGE_CTRL output; Z_VENT_CTRL output; Z_ATR_CTRL output; PACE_GND_CTRL output; VENT_GND_CTRL output; ATR_GND_CTRL output; LOWER_RATE_LIMIT input; VENT_PULSE_AMPLITUDE input; VENT_PULSE_WIDTH input; ATR_PULSE_AMPLITUDE input; ATR_PULSE_WIDTH input; ARP input; VRP input; HYSTERESIS input; RATE_SMOOTHING input; mode input; ADAPTIVE_PACERATE input

== stateflow chart Simulink_Assignment2/Adaptive Pacing Subsystem1/Chart ==
  state ResetPaceRate
    entry:
    PaceRate = double(LRL)
  state UpdatePaceRateStep
    entry:
    if PaceRate > TargetPaceRate
    StepSize = double((PaceRate - TargetPaceRate) / (RVT* 60 * 1000))
    elseif PaceRate < TargetPaceRate
    StepSize = double((TargetPaceRate - PaceRate) / (RT * 1000))
    else
    PaceRate = PaceRate;
    StepSize = 0.0;
    end
  state IncreasePaceRate
    entry:
    if PaceRate < TargetPaceRate
    PaceRate = PaceRate + StepSize;
    end
  state DecreasePaceRate
    entry:
    if PaceRate > TargetPaceRate
    PaceRate = PaceRate - StepSize;
    end
  (default) -> ResetPaceRate
  ResetPaceRate -> UpdatePaceRateStep : [mode > 4]
  UpdatePaceRateStep -> ResetPaceRate [order 1] : [mode < 5]
  UpdatePaceRateStep -> IncreasePaceRate [order 3] : [PaceRate < TargetPaceRate]
  UpdatePaceRateStep -> DecreasePaceRate [order 2] : [PaceRate > TargetPaceRate]
  IncreasePaceRate -> UpdatePaceRateStep [order 1] : [PaceRate >= TargetPaceRate]
  DecreasePaceRate -> UpdatePaceRateStep [order 1] : [PaceRate <= TargetPaceRate]
  DecreasePaceRate -> DecreasePaceRate [order 2] : [after(1,msec)]
  IncreasePaceRate -> IncreasePaceRate [order 2] : [after(1,msec)]
  data: mode input; LRL input uint8; RVT input; TargetPaceRate input; RT input; PaceRate output; StepSize local

== stateflow chart Simulink_Assignment2/DCM Reciever/Chart ==
  settings: executeAtInitialization=1
  state SET_PARAM
    entry:
    mode = rxdata(3)
    LOWER_RATE_LIMIT = rxdata(4);
    UPPER_RATE_LIMIT = rxdata(5);
    ATR_PULSE_AMPLITUDE = typecast(rxdata(6:9), 'single');
    VENT_PULSE_AMPLITUDE = typecast(rxdata(10:13), 'single');
    ATR_PULSE_WIDTH = typecast(rxdata(14:17), 'single');
    VENT_PULSE_WIDTH = typecast(rxdata(18:21), 'single');
    VRP = typecast(rxdata(22:23), 'uint16');
    ARP = typecast(rxdata(24:25), 'uint16');
    HYSTERESIS = rxdata(26);
    RATE_SMOOTHING = rxdata(27);
    ACTIVITY_THRESHOLD = rxdata(28);
    REACTION_TIME = rxdata(29); % seconds
    RESPONSE_FACTOR = rxdata(30);
    RECOVERY_TIME = rxdata(31);
    send_params();
  state INITIAL
    %Set initial values of parameter
    mode = 9;
    LOWER_RATE_LIMIT = 60;
    UPPER_RATE_LIMIT = 120;
    ATR_PULSE_AMPLITUDE = 3.5;
    VENT_PULSE_AMPLITUDE = 3.5;
    ATR_PULSE_WIDTH = 0.4;
    VENT_PULSE_WIDTH = 0.4;
    VRP = 320;
    ARP = 250;
    HYSTERESIS = 1;
    RATE_SMOOTHING = 1;
    ACTIVITY_THRESHOLD = 4;
    REACTION_TIME = 30; % seconds
    RESPONSE_FACTOR = 8; %factor 1-16
    RECOVERY_TIME = 5; %s
  state STANDBY
  state ECHO_PARAM
    entry:
    send_params();
  SET_PARAM -> STANDBY
  (junction 12) -> SET_PARAM [order 2] : [rxdata(2) == hex2dec('55')]
  (default) -> INITIAL
  (junction 14) -> STANDBY [order 2]
  STANDBY -> (junction 14) : [status == 0]
  (junction 14) -> (junction 12) [order 1] : [rxdata(1) == hex2dec('16')]
  INITIAL -> STANDBY
  (junction 12) -> ECHO_PARAM [order 1] : [rxdata(2) == hex2dec('22')]
  ECHO_PARAM -> STANDBY
  data: mode output uint8; LOWER_RATE_LIMIT output uint8; UPPER_RATE_LIMIT output uint8; status input uint8; rxdata input uint8; ATR_PULSE_AMPLITUDE output single; VENT_PULSE_AMPLITUDE output single; ATR_PULSE_WIDTH output single; VENT_PULSE_WIDTH output single; VRP output uint16; ARP output uint16; HYSTERESIS output uint8; RATE_SMOOTHING output uint8; ACTIVITY_THRESHOLD output uint8; REACTION_TIME output uint8; RESPONSE_FACTOR output uint8; RECOVERY_TIME output uint8

== matlab function Simulink_Assignment2/Adaptive Pacing Subsystem1/MATLAB Function ==
  data: u input; avg output
function avg = movingAverage(u)
    % Persistent variables to store buffer and index
    persistent buffer index count;

    % Number of samples for 1-second average
    N = 20;

    % Initialize buffer and index on first call
    if isempty(buffer)
        buffer = zeros(1, N); % Circular buffer
        index = 1;            % Current write position
        count = 0;            % Number of values added
    end

    % Add new sample to the buffer
    buffer(index) = u;
    index = mod(index, N) + 1; % Update index (wraps around)

    % Update count of samples (max is N)
    count = min(count + 1, N);

    % Calculate average (sum only the valid elements)
    avg = sum(buffer) / count;
end

== matlab function Simulink_Assignment2/Adaptive Pacing Subsystem1/MATLAB Function1 ==
  data: AL input; TargetPaceRate output; LRL input; MSR input; RF input; AT input
function TargetPaceRate = CalculatePacingRate(AL, LRL, MSR, RF, AT)

    if AL < AT
        TargetPaceRate = LRL;
    else
        TargetPaceRate = min(LRL + (AL - AT) * RF, MSR);
    end
end
